simulink library "interfaccia"  (R2024b)
settings: Solver=VariableStepAuto  StartTime=0.0  StopTime=10.0  RelTol=1e-3
settings Model: Creator=mainuser  LastModifiedBy=mainuser

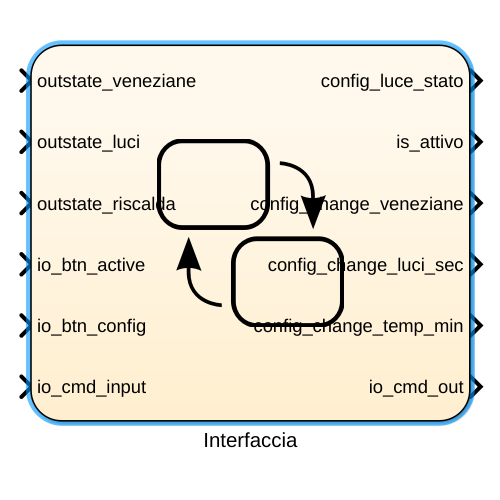
[thumbnail: Simulink's stored preview of the top-level diagram]
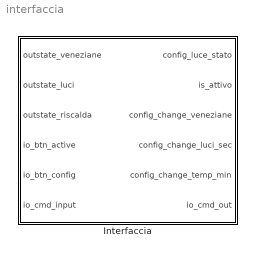
== system interfaccia ==
  Interfaccia : Stateflow chart  TreatAsAtomicUnit=on

== stateflow chart interfaccia/Interfaccia ==
  data: config_luce_stato output; is_attivo output; outstate_veneziane input; outstate_luci input; outstate_riscalda input; io_btn_active input; io_btn_config input; io_cmd_input input; config_change_veneziane output; config_change_luci_sec output; config_change_temp_min output; io_cmd_out output; config_set_mode local
